simulink model "tdoa_sim_signal_gen"  (R2024b)
settings: Solver=VariableStepAuto  StartTime=0.0  StopTime=100000  RelTol=1e-3
libraries: commanabbnd3 x1, dspfdesign x1, simulink x1
settings Model: Creator=LAB-win10  LastModifiedBy=LAB-win10

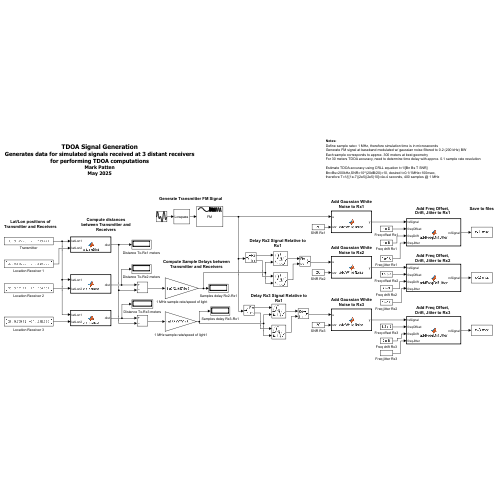
[thumbnail: Simulink's stored preview of the top-level diagram]
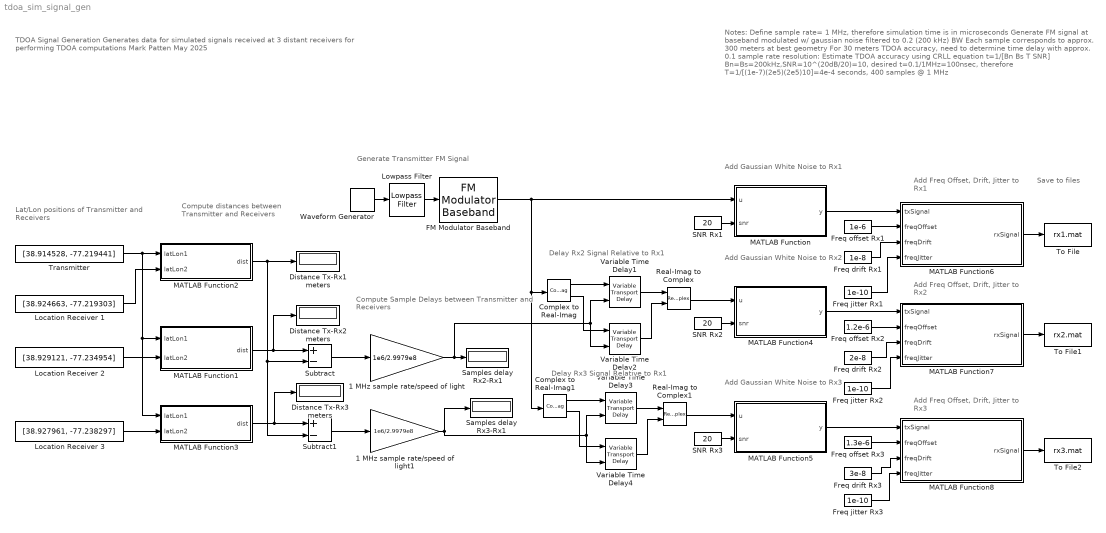
== system tdoa_sim_signal_gen ==
  note: Lat/Lon positions of Transmitter and Receivers
  note: TDOA Signal Generation
      | Generates data for simulated signals received at 3 distant receivers for performing TDOA computations
      | Mark Patten
      | May 2025
  note: Compute distances between Transmitter and Receivers
  note: Generate Transmitter FM Signal
  note: Compute Sample Delays between Transmitter and Receivers
  note: Delay Rx2 Signal Relative to Rx1
  note: Delay Rx3 Signal Relative to Rx1
  note: Add Gaussian White Noise to Rx1
  note: Add Gaussian White Noise to Rx2
  note: Add Gaussian White Noise to Rx3
  note: Add Freq Offset, Drift, Jitter to Rx1
  note: Add Freq Offset, Drift, Jitter to Rx2
  note: Add Freq Offset, Drift, Jitter to Rx3
  note: Save to files
  note: Notes:
      | Define sample rate= 1 MHz, therefore simulation time is in microseconds
      | Generate FM signal at baseband modulated w/ gaussian noise filtered to 0.2 (200 kHz) BW
      | Each sample corresponds to approx. 300 meters at best geometry
      | For 30 meters TDOA accuracy, need to determine time delay with approx. 0.1 sample rate resolution:
      |
      | Estimate TDOA accuracy using CRLL equation t=1/[Bn Bs T SNR]
      | Bn=Bs=200kHz,SNR=10^(20dB/20)=10, desired t=0.1/1MHz=100nsec,
      | therefore T=1/[(1e-7)(2e5)(2e5)10]=4e-4 seconds, 400 samples @ 1 MHz
  1 MHz sample rate/speed of light : Gain  Gain=1e6/2.9979e8
  1 MHz sample rate/speed of light1 : Gain  Gain=1e6/2.9979e8
  Complex to Real-Imag : ComplexToRealImag
  Complex to Real-Imag1 : ComplexToRealImag
  Distance Tx-Rx1 meters : Display
  Distance Tx-Rx2 meters : Display
  Distance Tx-Rx3 meters : Display
  FM Modulator Baseband : commanabbnd3/FM Modulator Baseband  FrequencyDeviation=.1  SimulateUsing=Code generation
  Freq drift Rx1 : Constant  Value=1e-8
  Freq drift Rx2 : Constant  Value=2e-8
  Freq drift Rx3 : Constant  Value=3e-8
  Freq jitter Rx1 : Constant  Value=1e-10
  Freq jitter Rx2 : Constant  Value=1e-10
  Freq jitter Rx3 : Constant  Value=1e-10
  Freq offset Rx1 : Constant  Value=1e-6
  Freq offset Rx2 : Constant  Value=1.2e-6
  Freq offset Rx3 : Constant  Value=1.3e-6
  Location Receiver 1 : Constant  Value=[38.924663, -77.219303]
  Location Receiver 2 : Constant  Value=[38.929121, -77.234954]
  Location Receiver 3 : Constant  Value=[38.927961, -77.238297]
  Lowpass Filter : dspfdesign/Lowpass Filter  FilterType=FIR  DesignForMinimumOrder=on  FilterOrder=50  PassbandFrequency=0.2  StopbandFrequency=0.5  PassbandRipple=3  StopbandAttenuation=40  SampleRateMode=Use normalized frequency (0 to 1)  SampleRate=44100  SimulateUsing=Interpreted execution  roundingMode=Floor  coeffsDataTypeStr=fixdt(1,16)
  MATLAB Function : MATLAB Function  TreatAsAtomicUnit=on
  MATLAB Function1 : MATLAB Function  TreatAsAtomicUnit=on
  MATLAB Function2 : MATLAB Function  TreatAsAtomicUnit=on
  MATLAB Function3 : MATLAB Function  TreatAsAtomicUnit=on
  MATLAB Function4 : MATLAB Function  TreatAsAtomicUnit=on
  MATLAB Function5 : MATLAB Function  TreatAsAtomicUnit=on
  MATLAB Function6 : MATLAB Function  TreatAsAtomicUnit=on
  MATLAB Function7 : MATLAB Function  TreatAsAtomicUnit=on
  MATLAB Function8 : MATLAB Function  TreatAsAtomicUnit=on
  Real-Imag to Complex : RealImagToComplex
  Real-Imag to Complex1 : RealImagToComplex
  SNR Rx1 : Constant  Value=20
  SNR Rx2 : Constant  Value=20
  SNR Rx3 : Constant  Value=20
  Samples delay Rx2-Rx1 : Display
  Samples delay Rx3-Rx1 : Display
  Subtract : Sum  Inputs=+-
  Subtract1 : Sum  Inputs=+-
  To File : ToFile  Filename=rx1.mat  SaveFormat=Timeseries
  To File1 : ToFile  Filename=rx2.mat  SaveFormat=Timeseries
  To File2 : ToFile  Filename=rx3.mat  SaveFormat=Timeseries
  Transmitter : Constant  Value=[38.914528, -77.219441]
  Variable Time Delay{1..4} (4 alike) : VariableTransportDelay  MaximumDelay=10
  Waveform Generator : simulink/Sources/Waveform Generator  OutMin=[]  OutMax=[]  OutDataTypeStr=double  SelectedSignal=1  Signals=gaussian(0,1,.417)####  BlockNames=MultiportSwitch_43672fd25cd341a#MultiportSwitch_8ac560371fde4a7#MultiportSwitch_875f254c7bc84f0#MultiportSwitch_c6db4b3ef64c4ac#MultiportSwitch_4dd9d8b26afc496  SampleTime=1
  wires:
  Waveform Generator/1 -> Lowpass Filter/1
  Lowpass Filter/1 -> FM Modulator Baseband/1
  Complex to Real-Imag/2 -> Variable Time Delay2/1
  1 MHz sample rate/speed of light/1 -> Variable Time Delay1/2, Variable Time Delay2/2, Samples delay Rx2-Rx1/1
  Variable Time Delay1/1 -> Real-Imag to Complex/1
  Complex to Real-Imag/1 -> Variable Time Delay1/1
  Variable Time Delay2/1 -> Real-Imag to Complex/2
  MATLAB Function2/1(dist) -> Subtract1/2, Subtract/2, Distance Tx-Rx1 meters/1
  Location Receiver 1/1 -> MATLAB Function2/2(latLon2)
  Location Receiver 2/1 -> MATLAB Function1/2(latLon2)
  Location Receiver 3/1 -> MATLAB Function3/2(latLon2)
  MATLAB Function1/1(dist) -> Subtract/1, Distance Tx-Rx2 meters/1
  Transmitter/1 -> MATLAB Function3/1(latLon1), MATLAB Function1/1(latLon1), MATLAB Function2/1(latLon1)
  1 MHz sample rate/speed of light1/1 -> Variable Time Delay4/2, Variable Time Delay3/2, Samples delay Rx3-Rx1/1
  Complex to Real-Imag1/2 -> Variable Time Delay4/1
  FM Modulator Baseband/1 -> Complex to Real-Imag1/1, Complex to Real-Imag/1, MATLAB Function/1(u)
  Variable Time Delay4/1 -> Real-Imag to Complex1/2
  Complex to Real-Imag1/1 -> Variable Time Delay3/1
  Variable Time Delay3/1 -> Real-Imag to Complex1/1
  MATLAB Function3/1(dist) -> Subtract1/1, Distance Tx-Rx3 meters/1
  Subtract1/1 -> 1 MHz sample rate/speed of light1/1
  Subtract/1 -> 1 MHz sample rate/speed of light/1
  SNR Rx1/1 -> MATLAB Function/2(snr)
  SNR Rx2/1 -> MATLAB Function4/2(snr)
  Real-Imag to Complex/1 -> MATLAB Function4/1(u)
  SNR Rx3/1 -> MATLAB Function5/2(snr)
  Real-Imag to Complex1/1 -> MATLAB Function5/1(u)
  MATLAB Function/1(y) -> MATLAB Function6/1(txSignal)
  MATLAB Function4/1(y) -> MATLAB Function7/1(txSignal)
  MATLAB Function5/1(y) -> MATLAB Function8/1(txSignal)
  Freq offset Rx1/1 -> MATLAB Function6/2(freqOffset)
  Freq drift Rx1/1 -> MATLAB Function6/3(freqDrift)
  Freq jitter Rx1/1 -> MATLAB Function6/4(freqJitter)
  Freq jitter Rx2/1 -> MATLAB Function7/4(freqJitter)
  Freq drift Rx2/1 -> MATLAB Function7/3(freqDrift)
  Freq offset Rx2/1 -> MATLAB Function7/2(freqOffset)
  Freq jitter Rx3/1 -> MATLAB Function8/4(freqJitter)
  Freq drift Rx3/1 -> MATLAB Function8/3(freqDrift)
  Freq offset Rx3/1 -> MATLAB Function8/2(freqOffset)
  MATLAB Function6/1(rxSignal) -> To File/1
  MATLAB Function7/1(rxSignal) -> To File1/1
  MATLAB Function8/1(rxSignal) -> To File2/1

== matlab function tdoa_sim_signal_gen/MATLAB Function1 ==
  data: latLon1 input; dist output; latLon2 input
function dist = latLonDist(latLon1,latLon2)
% dist = latLonDist(latLon1,latLon2)
% distance between two latitude/longitute positions in meters

avgLat = (latLon1(1) + latLon2(1))/2;
earthCirc = 24901.55 * 5280 * 12 * 2.54 / 100;
distx = cosd(avgLat) * (latLon2(2) - latLon1(2)) * earthCirc / 360;
disty = (latLon2(1) - latLon1(1)) * earthCirc / 360;
dist = (distx^2 + disty^2)^0.5;

== matlab function tdoa_sim_signal_gen/MATLAB Function3 ==
  data: latLon1 input; dist output; latLon2 input
function dist = latLonDist(latLon1,latLon2)
% dist = latLonDist(latLon1,latLon2)
% distance between two latitude/longitute positions in meters

avgLat = (latLon1(1) + latLon2(1))/2;
earthCirc = 24901.55 * 5280 * 12 * 2.54 / 100;
distx = cosd(avgLat) * (latLon2(2) - latLon1(2)) * earthCirc / 360;
disty = (latLon2(1) - latLon1(1)) * earthCirc / 360;
dist = (distx^2 + disty^2)^0.5;

== matlab function tdoa_sim_signal_gen/MATLAB Function2 ==
  data: latLon1 input; dist output; latLon2 input
function dist = latLonDist(latLon1,latLon2)
% dist = latLonDist(latLon1,latLon2)
% distance between two latitude/longitute positions in meters

avgLat = (latLon1(1) + latLon2(1))/2;
earthCirc = 24901.55 * 5280 * 12 * 2.54 / 100;
distx = cosd(avgLat) * (latLon2(2) - latLon1(2)) * earthCirc / 360;
disty = (latLon2(1) - latLon1(1)) * earthCirc / 360;
dist = (distx^2 + disty^2)^0.5;

== matlab function tdoa_sim_signal_gen/MATLAB Function ==
  data: u input; y output; snr input
function y = addWhiteNoise(u,snr)

y = u+randn(size(u))*(10^(snr/10));

== matlab function tdoa_sim_signal_gen/MATLAB Function4 ==
  data: u input; y output; snr input
function y = addWhiteNoise(u,snr)

y = u+randn(size(u))*(10^(snr/10));

== matlab function tdoa_sim_signal_gen/MATLAB Function5 ==
  data: u input; y output; snr input
function y = addWhiteNoise(u,snr)

y = u+randn(size(u))*(10^(snr/10));

== matlab function tdoa_sim_signal_gen/MATLAB Function6 ==
  data: txSignal input; rxSignal output; freqOffset input; freqDrift input; freqJitter input
function rxSignal = addFreqDriftJitter(txSignal,freqOffset,freqDrift,freqJitter)
% function rxSignal = addFreqDriftJitter(txSignal,freqOffset,freqDrift,freqJitter)
%
% Simulates effects of imperfect receiver reference oscillators, causing frequency offset, drift, and jitter
% rxSignal --- output signal with added frequency offset, drift, and jitter
% r% txSignal --- input signal
% freqOffset --- frequency offset (two receiver LOs may be typically 10-6 of each other, so use that) 
% freqDrift --- frequency drift (say, 100 times less than offset, so use 10-8)
% freqJitter ---- random noise frequency in frequency (say, 100 times less than drift, so use 10-10)
rxSignal = txSignal;
phaseDrift=0;
for i=1:length(txSignal)
    rxSignal(i) = rxSignal(i) * cos(2*pi*phaseDrift)+i+sin(2*pi*phaseDrift);
    phaseDrift=phaseDrift+freqOffset;
    freqOffset=freqOffset+freqDrift+freqJitter*randn(1);
end

== matlab function tdoa_sim_signal_gen/MATLAB Function7 ==
  data: txSignal input; rxSignal output; freqOffset input; freqDrift input; freqJitter input
function rxSignal = addFreqDriftJitter(txSignal,freqOffset,freqDrift,freqJitter)
% function rxSignal = addFreqDriftJitter(txSignal,freqOffset,freqDrift,freqJitter)
%
% Simulates effects of imperfect receiver reference oscillators, causing frequency offset, drift, and jitter
% rxSignal --- output signal with added frequency offset, drift, and jitter
% r% txSignal --- input signal
% freqOffset --- frequency offset (two receiver LOs may be typically 10-6 of each other, so use that) 
% freqDrift --- frequency drift (say, 100 times less than offset, so use 10-8)
% freqJitter ---- random noise frequency in frequency (say, 100 times less than drift, so use 10-10)
rxSignal = txSignal;
phaseDrift=0;
for i=1:length(txSignal)
    rxSignal(i) = rxSignal(i) * cos(2*pi*phaseDrift)+i+sin(2*pi*phaseDrift);
    phaseDrift=phaseDrift+freqOffset;
    freqOffset=freqOffset+freqDrift+freqJitter*randn(1);
end

== matlab function tdoa_sim_signal_gen/MATLAB Function8 ==
  data: txSignal input; rxSignal output; freqOffset input; freqDrift input; freqJitter input
function rxSignal = addFreqDriftJitter(txSignal,freqOffset,freqDrift,freqJitter)
% function rxSignal = addFreqDriftJitter(txSignal,freqOffset,freqDrift,freqJitter)
%
% Simulates effects of imperfect receiver reference oscillators, causing frequency offset, drift, and jitter
% rxSignal --- output signal with added frequency offset, drift, and jitter
% r% txSignal --- input signal
% freqOffset --- frequency offset (two receiver LOs may be typically 10-6 of each other, so use that) 
% freqDrift --- frequency drift (say, 100 times less than offset, so use 10-8)
% freqJitter ---- random noise frequency in frequency (say, 100 times less than drift, so use 10-10)
rxSignal = txSignal;
phaseDrift=0;
for i=1:length(txSignal)
    rxSignal(i) = rxSignal(i) * cos(2*pi*phaseDrift)+i+sin(2*pi*phaseDrift);
    phaseDrift=phaseDrift+freqOffset;
    freqOffset=freqOffset+freqDrift+freqJitter*randn(1);
end
